simulink model "MdXX_DoneChk"  (R2024b)
settings: Solver=FixedStepDiscrete  StartTime=0.0  StopTime=10.0  FixedStep=0.01  RelTol=1e-3
undefined symbols (not defined in the file or in its folder): KeSMSuVehicleModelConfig_Val
libraries: simulink x44
(part 3 of 3)

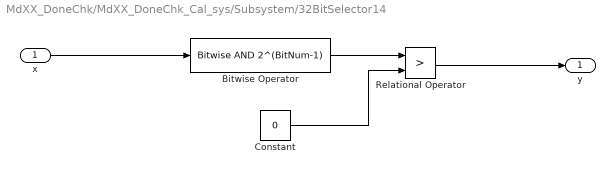
== system MdXX_DoneChk/MdXX_DoneChk_Cal_sys/Subsystem/32BitSelector14 ==
  x : Inport
  Bitwise Operator : simulink/Logic and Bit Operations/Bitwise Operator  logicop=AND  UseBitMask=on  BitMask=2^(BitNum-1)  BitMaskRealWorld=Stored Integer
  Constant : Constant  Value=0  OutDataTypeStr=uint32
  Relational Operator : RelationalOperator  Operator=>  OutDataTypeStr=boolean  RndMeth=Simplest  InputSameDT=off
  y : Outport  VectorParamsAs1DForOutWhenUnconnected=off
  wires:
  Relational Operator/1 -> y/1
  Constant/1 -> Relational Operator/2
  x/1 -> Bitwise Operator/1
  Bitwise Operator/1 -> Relational Operator/1

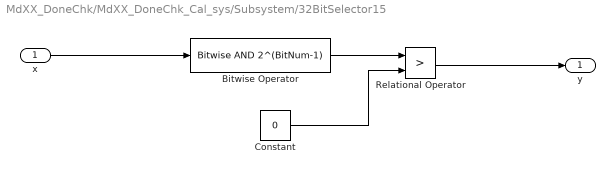
== system MdXX_DoneChk/MdXX_DoneChk_Cal_sys/Subsystem/32BitSelector15 ==
  x : Inport
  Bitwise Operator : simulink/Logic and Bit Operations/Bitwise Operator  logicop=AND  UseBitMask=on  BitMask=2^(BitNum-1)  BitMaskRealWorld=Stored Integer
  Constant : Constant  Value=0  OutDataTypeStr=uint32
  Relational Operator : RelationalOperator  Operator=>  OutDataTypeStr=boolean  RndMeth=Simplest  InputSameDT=off
  y : Outport  VectorParamsAs1DForOutWhenUnconnected=off
  wires:
  Bitwise Operator/1 -> Relational Operator/1
  x/1 -> Bitwise Operator/1
  Constant/1 -> Relational Operator/2
  Relational Operator/1 -> y/1

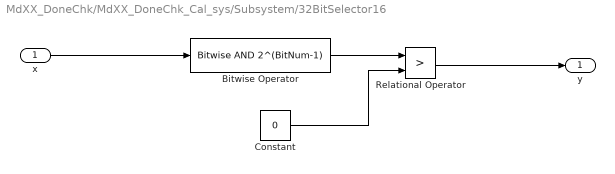
== system MdXX_DoneChk/MdXX_DoneChk_Cal_sys/Subsystem/32BitSelector16 ==
  x : Inport
  Bitwise Operator : simulink/Logic and Bit Operations/Bitwise Operator  logicop=AND  UseBitMask=on  BitMask=2^(BitNum-1)  BitMaskRealWorld=Stored Integer
  Constant : Constant  Value=0  OutDataTypeStr=uint32
  Relational Operator : RelationalOperator  Operator=>  OutDataTypeStr=boolean  RndMeth=Simplest  InputSameDT=off
  y : Outport  VectorParamsAs1DForOutWhenUnconnected=off
  wires:
  Relational Operator/1 -> y/1
  Constant/1 -> Relational Operator/2
  x/1 -> Bitwise Operator/1
  Bitwise Operator/1 -> Relational Operator/1

== system MdXX_DoneChk/MdXX_DoneChk_Cal_sys/Subsystem/32BitSelector17 ==
  x : Inport
  Bitwise Operator : simulink/Logic and Bit Operations/Bitwise Operator  logicop=AND  UseBitMask=on  BitMask=2^(BitNum-1)  BitMaskRealWorld=Stored Integer
  Constant : Constant  Value=0  OutDataTypeStr=uint32
  Relational Operator : RelationalOperator  Operator=>  OutDataTypeStr=boolean  RndMeth=Simplest  InputSameDT=off
  y : Outport  VectorParamsAs1DForOutWhenUnconnected=off
  wires:
  Bitwise Operator/1 -> Relational Operator/1
  x/1 -> Bitwise Operator/1
  Constant/1 -> Relational Operator/2
  Relational Operator/1 -> y/1

== system MdXX_DoneChk/MdXX_DoneChk_Cal_sys/Subsystem/32BitSelector18 ==
  x : Inport
  Bitwise Operator : simulink/Logic and Bit Operations/Bitwise Operator  logicop=AND  UseBitMask=on  BitMask=2^(BitNum-1)  BitMaskRealWorld=Stored Integer
  Constant : Constant  Value=0  OutDataTypeStr=uint32
  Relational Operator : RelationalOperator  Operator=>  OutDataTypeStr=boolean  RndMeth=Simplest  InputSameDT=off
  y : Outport  VectorParamsAs1DForOutWhenUnconnected=off
  wires:
  Relational Operator/1 -> y/1
  Constant/1 -> Relational Operator/2
  x/1 -> Bitwise Operator/1
  Bitwise Operator/1 -> Relational Operator/1

== system MdXX_DoneChk/MdXX_DoneChk_Cal_sys/Subsystem/32BitSelector19 ==
  x : Inport
  Bitwise Operator : simulink/Logic and Bit Operations/Bitwise Operator  logicop=AND  UseBitMask=on  BitMask=2^(BitNum-1)  BitMaskRealWorld=Stored Integer
  Constant : Constant  Value=0  OutDataTypeStr=uint32
  Relational Operator : RelationalOperator  Operator=>  OutDataTypeStr=boolean  RndMeth=Simplest  InputSameDT=off
  y : Outport  VectorParamsAs1DForOutWhenUnconnected=off
  wires:
  Bitwise Operator/1 -> Relational Operator/1
  x/1 -> Bitwise Operator/1
  Constant/1 -> Relational Operator/2
  Relational Operator/1 -> y/1

== system MdXX_DoneChk/MdXX_DoneChk_Cal_sys/Subsystem/32BitSelector2 ==
  x : Inport
  Bitwise Operator : simulink/Logic and Bit Operations/Bitwise Operator  logicop=AND  UseBitMask=on  BitMask=2^(BitNum-1)  BitMaskRealWorld=Stored Integer
  Constant : Constant  Value=0  OutDataTypeStr=uint32
  Relational Operator : RelationalOperator  Operator=>  OutDataTypeStr=boolean  RndMeth=Simplest  InputSameDT=off
  y : Outport  VectorParamsAs1DForOutWhenUnconnected=off
  wires:
  Relational Operator/1 -> y/1
  Constant/1 -> Relational Operator/2
  x/1 -> Bitwise Operator/1
  Bitwise Operator/1 -> Relational Operator/1

== system MdXX_DoneChk/MdXX_DoneChk_Cal_sys/Subsystem/32BitSelector20 ==
  x : Inport
  Bitwise Operator : simulink/Logic and Bit Operations/Bitwise Operator  logicop=AND  UseBitMask=on  BitMask=2^(BitNum-1)  BitMaskRealWorld=Stored Integer
  Constant : Constant  Value=0  OutDataTypeStr=uint32
  Relational Operator : RelationalOperator  Operator=>  OutDataTypeStr=boolean  RndMeth=Simplest  InputSameDT=off
  y : Outport  VectorParamsAs1DForOutWhenUnconnected=off
  wires:
  Relational Operator/1 -> y/1
  Constant/1 -> Relational Operator/2
  x/1 -> Bitwise Operator/1
  Bitwise Operator/1 -> Relational Operator/1

== system MdXX_DoneChk/MdXX_DoneChk_Cal_sys/Subsystem/32BitSelector21 ==
  x : Inport
  Bitwise Operator : simulink/Logic and Bit Operations/Bitwise Operator  logicop=AND  UseBitMask=on  BitMask=2^(BitNum-1)  BitMaskRealWorld=Stored Integer
  Constant : Constant  Value=0  OutDataTypeStr=uint32
  Relational Operator : RelationalOperator  Operator=>  OutDataTypeStr=boolean  RndMeth=Simplest  InputSameDT=off
  y : Outport  VectorParamsAs1DForOutWhenUnconnected=off
  wires:
  Bitwise Operator/1 -> Relational Operator/1
  x/1 -> Bitwise Operator/1
  Constant/1 -> Relational Operator/2
  Relational Operator/1 -> y/1

== system MdXX_DoneChk/MdXX_DoneChk_Cal_sys/Subsystem/32BitSelector22 ==
  x : Inport
  Bitwise Operator : simulink/Logic and Bit Operations/Bitwise Operator  logicop=AND  UseBitMask=on  BitMask=2^(BitNum-1)  BitMaskRealWorld=Stored Integer
  Constant : Constant  Value=0  OutDataTypeStr=uint32
  Relational Operator : RelationalOperator  Operator=>  OutDataTypeStr=boolean  RndMeth=Simplest  InputSameDT=off
  y : Outport  VectorParamsAs1DForOutWhenUnconnected=off
  wires:
  Relational Operator/1 -> y/1
  Constant/1 -> Relational Operator/2
  x/1 -> Bitwise Operator/1
  Bitwise Operator/1 -> Relational Operator/1

== system MdXX_DoneChk/MdXX_DoneChk_Cal_sys/Subsystem/32BitSelector23 ==
  x : Inport
  Bitwise Operator : simulink/Logic and Bit Operations/Bitwise Operator  logicop=AND  UseBitMask=on  BitMask=2^(BitNum-1)  BitMaskRealWorld=Stored Integer
  Constant : Constant  Value=0  OutDataTypeStr=uint32
  Relational Operator : RelationalOperator  Operator=>  OutDataTypeStr=boolean  RndMeth=Simplest  InputSameDT=off
  y : Outport  VectorParamsAs1DForOutWhenUnconnected=off
  wires:
  Bitwise Operator/1 -> Relational Operator/1
  x/1 -> Bitwise Operator/1
  Constant/1 -> Relational Operator/2
  Relational Operator/1 -> y/1

== system MdXX_DoneChk/MdXX_DoneChk_Cal_sys/Subsystem/32BitSelector24 ==
  x : Inport
  Bitwise Operator : simulink/Logic and Bit Operations/Bitwise Operator  logicop=AND  UseBitMask=on  BitMask=2^(BitNum-1)  BitMaskRealWorld=Stored Integer
  Constant : Constant  Value=0  OutDataTypeStr=uint32
  Relational Operator : RelationalOperator  Operator=>  OutDataTypeStr=boolean  RndMeth=Simplest  InputSameDT=off
  y : Outport  VectorParamsAs1DForOutWhenUnconnected=off
  wires:
  Relational Operator/1 -> y/1
  Constant/1 -> Relational Operator/2
  x/1 -> Bitwise Operator/1
  Bitwise Operator/1 -> Relational Operator/1

== system MdXX_DoneChk/MdXX_DoneChk_Cal_sys/Subsystem/32BitSelector25 ==
  x : Inport
  Bitwise Operator : simulink/Logic and Bit Operations/Bitwise Operator  logicop=AND  UseBitMask=on  BitMask=2^(BitNum-1)  BitMaskRealWorld=Stored Integer
  Constant : Constant  Value=0  OutDataTypeStr=uint32
  Relational Operator : RelationalOperator  Operator=>  OutDataTypeStr=boolean  RndMeth=Simplest  InputSameDT=off
  y : Outport  VectorParamsAs1DForOutWhenUnconnected=off
  wires:
  Bitwise Operator/1 -> Relational Operator/1
  x/1 -> Bitwise Operator/1
  Constant/1 -> Relational Operator/2
  Relational Operator/1 -> y/1

== system MdXX_DoneChk/MdXX_DoneChk_Cal_sys/Subsystem/32BitSelector26 ==
  x : Inport
  Bitwise Operator : simulink/Logic and Bit Operations/Bitwise Operator  logicop=AND  UseBitMask=on  BitMask=2^(BitNum-1)  BitMaskRealWorld=Stored Integer
  Constant : Constant  Value=0  OutDataTypeStr=uint32
  Relational Operator : RelationalOperator  Operator=>  OutDataTypeStr=boolean  RndMeth=Simplest  InputSameDT=off
  y : Outport  VectorParamsAs1DForOutWhenUnconnected=off
  wires:
  Relational Operator/1 -> y/1
  Constant/1 -> Relational Operator/2
  x/1 -> Bitwise Operator/1
  Bitwise Operator/1 -> Relational Operator/1

== system MdXX_DoneChk/MdXX_DoneChk_Cal_sys/Subsystem/32BitSelector27 ==
  x : Inport
  Bitwise Operator : simulink/Logic and Bit Operations/Bitwise Operator  logicop=AND  UseBitMask=on  BitMask=2^(BitNum-1)  BitMaskRealWorld=Stored Integer
  Constant : Constant  Value=0  OutDataTypeStr=uint32
  Relational Operator : RelationalOperator  Operator=>  OutDataTypeStr=boolean  RndMeth=Simplest  InputSameDT=off
  y : Outport  VectorParamsAs1DForOutWhenUnconnected=off
  wires:
  Bitwise Operator/1 -> Relational Operator/1
  x/1 -> Bitwise Operator/1
  Constant/1 -> Relational Operator/2
  Relational Operator/1 -> y/1

== system MdXX_DoneChk/MdXX_DoneChk_Cal_sys/Subsystem/32BitSelector28 ==
  x : Inport
  Bitwise Operator : simulink/Logic and Bit Operations/Bitwise Operator  logicop=AND  UseBitMask=on  BitMask=2^(BitNum-1)  BitMaskRealWorld=Stored Integer
  Constant : Constant  Value=0  OutDataTypeStr=uint32
  Relational Operator : RelationalOperator  Operator=>  OutDataTypeStr=boolean  RndMeth=Simplest  InputSameDT=off
  y : Outport  VectorParamsAs1DForOutWhenUnconnected=off
  wires:
  Relational Operator/1 -> y/1
  Constant/1 -> Relational Operator/2
  x/1 -> Bitwise Operator/1
  Bitwise Operator/1 -> Relational Operator/1

== system MdXX_DoneChk/MdXX_DoneChk_Cal_sys/Subsystem/32BitSelector29 ==
  x : Inport
  Bitwise Operator : simulink/Logic and Bit Operations/Bitwise Operator  logicop=AND  UseBitMask=on  BitMask=2^(BitNum-1)  BitMaskRealWorld=Stored Integer
  Constant : Constant  Value=0  OutDataTypeStr=uint32
  Relational Operator : RelationalOperator  Operator=>  OutDataTypeStr=boolean  RndMeth=Simplest  InputSameDT=off
  y : Outport  VectorParamsAs1DForOutWhenUnconnected=off
  wires:
  Bitwise Operator/1 -> Relational Operator/1
  x/1 -> Bitwise Operator/1
  Constant/1 -> Relational Operator/2
  Relational Operator/1 -> y/1

== system MdXX_DoneChk/MdXX_DoneChk_Cal_sys/Subsystem/32BitSelector3 ==
  x : Inport
  Bitwise Operator : simulink/Logic and Bit Operations/Bitwise Operator  logicop=AND  UseBitMask=on  BitMask=2^(BitNum-1)  BitMaskRealWorld=Stored Integer
  Constant : Constant  Value=0  OutDataTypeStr=uint32
  Relational Operator : RelationalOperator  Operator=>  OutDataTypeStr=boolean  RndMeth=Simplest  InputSameDT=off
  y : Outport  VectorParamsAs1DForOutWhenUnconnected=off
  wires:
  Bitwise Operator/1 -> Relational Operator/1
  x/1 -> Bitwise Operator/1
  Constant/1 -> Relational Operator/2
  Relational Operator/1 -> y/1

== system MdXX_DoneChk/MdXX_DoneChk_Cal_sys/Subsystem/32BitSelector30 ==
  x : Inport
  Bitwise Operator : simulink/Logic and Bit Operations/Bitwise Operator  logicop=AND  UseBitMask=on  BitMask=2^(BitNum-1)  BitMaskRealWorld=Stored Integer
  Constant : Constant  Value=0  OutDataTypeStr=uint32
  Relational Operator : RelationalOperator  Operator=>  OutDataTypeStr=boolean  RndMeth=Simplest  InputSameDT=off
  y : Outport  VectorParamsAs1DForOutWhenUnconnected=off
  wires:
  Relational Operator/1 -> y/1
  Constant/1 -> Relational Operator/2
  x/1 -> Bitwise Operator/1
  Bitwise Operator/1 -> Relational Operator/1

== system MdXX_DoneChk/MdXX_DoneChk_Cal_sys/Subsystem/32BitSelector31 ==
  x : Inport
  Bitwise Operator : simulink/Logic and Bit Operations/Bitwise Operator  logicop=AND  UseBitMask=on  BitMask=2^(BitNum-1)  BitMaskRealWorld=Stored Integer
  Constant : Constant  Value=0  OutDataTypeStr=uint32
  Relational Operator : RelationalOperator  Operator=>  OutDataTypeStr=boolean  RndMeth=Simplest  InputSameDT=off
  y : Outport  VectorParamsAs1DForOutWhenUnconnected=off
  wires:
  Relational Operator/1 -> y/1
  Constant/1 -> Relational Operator/2
  x/1 -> Bitwise Operator/1
  Bitwise Operator/1 -> Relational Operator/1

== system MdXX_DoneChk/MdXX_DoneChk_Cal_sys/Subsystem/32BitSelector32 ==
  x : Inport
  Bitwise Operator : simulink/Logic and Bit Operations/Bitwise Operator  logicop=AND  UseBitMask=on  BitMask=2^(BitNum-1)  BitMaskRealWorld=Stored Integer
  Constant : Constant  Value=0  OutDataTypeStr=uint32
  Relational Operator : RelationalOperator  Operator=>  OutDataTypeStr=boolean  RndMeth=Simplest  InputSameDT=off
  y : Outport  VectorParamsAs1DForOutWhenUnconnected=off
  wires:
  Relational Operator/1 -> y/1
  Constant/1 -> Relational Operator/2
  x/1 -> Bitwise Operator/1
  Bitwise Operator/1 -> Relational Operator/1

== system MdXX_DoneChk/MdXX_DoneChk_Cal_sys/Subsystem/32BitSelector33 ==
  x : Inport
  Bitwise Operator : simulink/Logic and Bit Operations/Bitwise Operator  logicop=AND  UseBitMask=on  BitMask=2^(BitNum-1)  BitMaskRealWorld=Stored Integer
  Constant : Constant  Value=0  OutDataTypeStr=uint32
  Relational Operator : RelationalOperator  Operator=>  OutDataTypeStr=boolean  RndMeth=Simplest  InputSameDT=off
  y : Outport  VectorParamsAs1DForOutWhenUnconnected=off
  wires:
  Bitwise Operator/1 -> Relational Operator/1
  x/1 -> Bitwise Operator/1
  Constant/1 -> Relational Operator/2
  Relational Operator/1 -> y/1

== system MdXX_DoneChk/MdXX_DoneChk_Cal_sys/Subsystem/32BitSelector34 ==
  x : Inport
  Bitwise Operator : simulink/Logic and Bit Operations/Bitwise Operator  logicop=AND  UseBitMask=on  BitMask=2^(BitNum-1)  BitMaskRealWorld=Stored Integer
  Constant : Constant  Value=0  OutDataTypeStr=uint32
  Relational Operator : RelationalOperator  Operator=>  OutDataTypeStr=boolean  RndMeth=Simplest  InputSameDT=off
  y : Outport  VectorParamsAs1DForOutWhenUnconnected=off
  wires:
  Relational Operator/1 -> y/1
  Constant/1 -> Relational Operator/2
  x/1 -> Bitwise Operator/1
  Bitwise Operator/1 -> Relational Operator/1

== system MdXX_DoneChk/MdXX_DoneChk_Cal_sys/Subsystem/32BitSelector35 ==
  x : Inport
  Bitwise Operator : simulink/Logic and Bit Operations/Bitwise Operator  logicop=AND  UseBitMask=on  BitMask=2^(BitNum-1)  BitMaskRealWorld=Stored Integer
  Constant : Constant  Value=0  OutDataTypeStr=uint32
  Relational Operator : RelationalOperator  Operator=>  OutDataTypeStr=boolean  RndMeth=Simplest  InputSameDT=off
  y : Outport  VectorParamsAs1DForOutWhenUnconnected=off
  wires:
  Bitwise Operator/1 -> Relational Operator/1
  x/1 -> Bitwise Operator/1
  Constant/1 -> Relational Operator/2
  Relational Operator/1 -> y/1

== system MdXX_DoneChk/MdXX_DoneChk_Cal_sys/Subsystem/32BitSelector36 ==
  x : Inport
  Bitwise Operator : simulink/Logic and Bit Operations/Bitwise Operator  logicop=AND  UseBitMask=on  BitMask=2^(BitNum-1)  BitMaskRealWorld=Stored Integer
  Constant : Constant  Value=0  OutDataTypeStr=uint32
  Relational Operator : RelationalOperator  Operator=>  OutDataTypeStr=boolean  RndMeth=Simplest  InputSameDT=off
  y : Outport  VectorParamsAs1DForOutWhenUnconnected=off
  wires:
  Bitwise Operator/1 -> Relational Operator/1
  x/1 -> Bitwise Operator/1
  Constant/1 -> Relational Operator/2
  Relational Operator/1 -> y/1

== system MdXX_DoneChk/MdXX_DoneChk_Cal_sys/Subsystem/32BitSelector37 ==
  x : Inport
  Bitwise Operator : simulink/Logic and Bit Operations/Bitwise Operator  logicop=AND  UseBitMask=on  BitMask=2^(BitNum-1)  BitMaskRealWorld=Stored Integer
  Constant : Constant  Value=0  OutDataTypeStr=uint32
  Relational Operator : RelationalOperator  Operator=>  OutDataTypeStr=boolean  RndMeth=Simplest  InputSameDT=off
  y : Outport  VectorParamsAs1DForOutWhenUnconnected=off
  wires:
  Relational Operator/1 -> y/1
  Constant/1 -> Relational Operator/2
  x/1 -> Bitwise Operator/1
  Bitwise Operator/1 -> Relational Operator/1

== system MdXX_DoneChk/MdXX_DoneChk_Cal_sys/Subsystem/32BitSelector38 ==
  x : Inport
  Bitwise Operator : simulink/Logic and Bit Operations/Bitwise Operator  logicop=AND  UseBitMask=on  BitMask=2^(BitNum-1)  BitMaskRealWorld=Stored Integer
  Constant : Constant  Value=0  OutDataTypeStr=uint32
  Relational Operator : RelationalOperator  Operator=>  OutDataTypeStr=boolean  RndMeth=Simplest  InputSameDT=off
  y : Outport  VectorParamsAs1DForOutWhenUnconnected=off
  wires:
  Bitwise Operator/1 -> Relational Operator/1
  x/1 -> Bitwise Operator/1
  Constant/1 -> Relational Operator/2
  Relational Operator/1 -> y/1

== system MdXX_DoneChk/MdXX_DoneChk_Cal_sys/Subsystem/32BitSelector39 ==
  x : Inport
  Bitwise Operator : simulink/Logic and Bit Operations/Bitwise Operator  logicop=AND  UseBitMask=on  BitMask=2^(BitNum-1)  BitMaskRealWorld=Stored Integer
  Constant : Constant  Value=0  OutDataTypeStr=uint32
  Relational Operator : RelationalOperator  Operator=>  OutDataTypeStr=boolean  RndMeth=Simplest  InputSameDT=off
  y : Outport  VectorParamsAs1DForOutWhenUnconnected=off
  wires:
  Bitwise Operator/1 -> Relational Operator/1
  x/1 -> Bitwise Operator/1
  Constant/1 -> Relational Operator/2
  Relational Operator/1 -> y/1

== system MdXX_DoneChk/MdXX_DoneChk_Cal_sys/Subsystem/32BitSelector4 ==
  x : Inport
  Bitwise Operator : simulink/Logic and Bit Operations/Bitwise Operator  logicop=AND  UseBitMask=on  BitMask=2^(BitNum-1)  BitMaskRealWorld=Stored Integer
  Constant : Constant  Value=0  OutDataTypeStr=uint32
  Relational Operator : RelationalOperator  Operator=>  OutDataTypeStr=boolean  RndMeth=Simplest  InputSameDT=off
  y : Outport  VectorParamsAs1DForOutWhenUnconnected=off
  wires:
  Relational Operator/1 -> y/1
  Constant/1 -> Relational Operator/2
  x/1 -> Bitwise Operator/1
  Bitwise Operator/1 -> Relational Operator/1

== system MdXX_DoneChk/MdXX_DoneChk_Cal_sys/Subsystem/32BitSelector5 ==
  x : Inport
  Bitwise Operator : simulink/Logic and Bit Operations/Bitwise Operator  logicop=AND  UseBitMask=on  BitMask=2^(BitNum-1)  BitMaskRealWorld=Stored Integer
  Constant : Constant  Value=0  OutDataTypeStr=uint32
  Relational Operator : RelationalOperator  Operator=>  OutDataTypeStr=boolean  RndMeth=Simplest  InputSameDT=off
  y : Outport  VectorParamsAs1DForOutWhenUnconnected=off
  wires:
  Bitwise Operator/1 -> Relational Operator/1
  x/1 -> Bitwise Operator/1
  Constant/1 -> Relational Operator/2
  Relational Operator/1 -> y/1

== system MdXX_DoneChk/MdXX_DoneChk_Cal_sys/Subsystem/32BitSelector6 ==
  x : Inport
  Bitwise Operator : simulink/Logic and Bit Operations/Bitwise Operator  logicop=AND  UseBitMask=on  BitMask=2^(BitNum-1)  BitMaskRealWorld=Stored Integer
  Constant : Constant  Value=0  OutDataTypeStr=uint32
  Relational Operator : RelationalOperator  Operator=>  OutDataTypeStr=boolean  RndMeth=Simplest  InputSameDT=off
  y : Outport  VectorParamsAs1DForOutWhenUnconnected=off
  wires:
  Relational Operator/1 -> y/1
  Constant/1 -> Relational Operator/2
  x/1 -> Bitwise Operator/1
  Bitwise Operator/1 -> Relational Operator/1

== system MdXX_DoneChk/MdXX_DoneChk_Cal_sys/Subsystem/32BitSelector7 ==
  x : Inport
  Bitwise Operator : simulink/Logic and Bit Operations/Bitwise Operator  logicop=AND  UseBitMask=on  BitMask=2^(BitNum-1)  BitMaskRealWorld=Stored Integer
  Constant : Constant  Value=0  OutDataTypeStr=uint32
  Relational Operator : RelationalOperator  Operator=>  OutDataTypeStr=boolean  RndMeth=Simplest  InputSameDT=off
  y : Outport  VectorParamsAs1DForOutWhenUnconnected=off
  wires:
  Bitwise Operator/1 -> Relational Operator/1
  x/1 -> Bitwise Operator/1
  Constant/1 -> Relational Operator/2
  Relational Operator/1 -> y/1

== system MdXX_DoneChk/MdXX_DoneChk_Cal_sys/Subsystem/32BitSelector8 ==
  x : Inport
  Bitwise Operator : simulink/Logic and Bit Operations/Bitwise Operator  logicop=AND  UseBitMask=on  BitMask=2^(BitNum-1)  BitMaskRealWorld=Stored Integer
  Constant : Constant  Value=0  OutDataTypeStr=uint32
  Relational Operator : RelationalOperator  Operator=>  OutDataTypeStr=boolean  RndMeth=Simplest  InputSameDT=off
  y : Outport  VectorParamsAs1DForOutWhenUnconnected=off
  wires:
  Relational Operator/1 -> y/1
  Constant/1 -> Relational Operator/2
  x/1 -> Bitwise Operator/1
  Bitwise Operator/1 -> Relational Operator/1

== system MdXX_DoneChk/MdXX_DoneChk_Cal_sys/Subsystem/32BitSelector9 ==
  x : Inport
  Bitwise Operator : simulink/Logic and Bit Operations/Bitwise Operator  logicop=AND  UseBitMask=on  BitMask=2^(BitNum-1)  BitMaskRealWorld=Stored Integer
  Constant : Constant  Value=0  OutDataTypeStr=uint32
  Relational Operator : RelationalOperator  Operator=>  OutDataTypeStr=boolean  RndMeth=Simplest  InputSameDT=off
  y : Outport  VectorParamsAs1DForOutWhenUnconnected=off
  wires:
  Bitwise Operator/1 -> Relational Operator/1
  x/1 -> Bitwise Operator/1
  Constant/1 -> Relational Operator/2
  Relational Operator/1 -> y/1

== system MdXX_DoneChk/MdXX_DoneChk_Cal_sys/Subsystem/Subsystem ==
  MdDone : Inport
  MdEn : Inport  Port=2
  Constant : Constant  Value=0  OutDataTypeStr=uint8
  Switch : Switch  Criteria=u2 > Threshold  SaturateOnIntegerOverflow=off  InputSameDT=off
  MdDoneOut : Outport  VectorParamsAs1DForOutWhenUnconnected=off
  wires:
  MdEn/1 -> Switch/2
  Switch/1 -> MdDoneOut/1
  MdDone/1 -> Switch/1
  Constant/1 -> Switch/3

== system MdXX_DoneChk/MdXX_DoneChk_Cal_sys/Subsystem/Subsystem1 ==
  MdDone : Inport
  MdEn : Inport  Port=2
  Constant : Constant  Value=0  OutDataTypeStr=uint8
  Switch : Switch  Criteria=u2 > Threshold  SaturateOnIntegerOverflow=off  InputSameDT=off
  MdDoneOut : Outport  VectorParamsAs1DForOutWhenUnconnected=off
  wires:
  Constant/1 -> Switch/3
  MdDone/1 -> Switch/1
  Switch/1 -> MdDoneOut/1
  MdEn/1 -> Switch/2

== system MdXX_DoneChk/MdXX_DoneChk_Cal_sys/Subsystem/Subsystem10 ==
  MdDone : Inport
  MdEn : Inport  Port=2
  Constant : Constant  Value=0  OutDataTypeStr=uint8
  Switch : Switch  Criteria=u2 > Threshold  SaturateOnIntegerOverflow=off  InputSameDT=off
  MdDoneOut : Outport  VectorParamsAs1DForOutWhenUnconnected=off
  wires:
  MdEn/1 -> Switch/2
  Switch/1 -> MdDoneOut/1
  MdDone/1 -> Switch/1
  Constant/1 -> Switch/3

== system MdXX_DoneChk/MdXX_DoneChk_Cal_sys/Subsystem/Subsystem11 ==
  MdDone : Inport
  MdEn : Inport  Port=2
  Constant : Constant  Value=0  OutDataTypeStr=uint8
  Switch : Switch  Criteria=u2 > Threshold  SaturateOnIntegerOverflow=off  InputSameDT=off
  MdDoneOut : Outport  VectorParamsAs1DForOutWhenUnconnected=off
  wires:
  Constant/1 -> Switch/3
  MdDone/1 -> Switch/1
  Switch/1 -> MdDoneOut/1
  MdEn/1 -> Switch/2

== system MdXX_DoneChk/MdXX_DoneChk_Cal_sys/Subsystem/Subsystem12 ==
  MdDone : Inport
  MdEn : Inport  Port=2
  Constant : Constant  Value=0  OutDataTypeStr=uint8
  Switch : Switch  Criteria=u2 > Threshold  SaturateOnIntegerOverflow=off  InputSameDT=off
  MdDoneOut : Outport  VectorParamsAs1DForOutWhenUnconnected=off
  wires:
  MdEn/1 -> Switch/2
  Switch/1 -> MdDoneOut/1
  MdDone/1 -> Switch/1
  Constant/1 -> Switch/3

== system MdXX_DoneChk/MdXX_DoneChk_Cal_sys/Subsystem/Subsystem13 ==
  MdDone : Inport
  MdEn : Inport  Port=2
  Constant : Constant  Value=0  OutDataTypeStr=uint8
  Switch : Switch  Criteria=u2 > Threshold  SaturateOnIntegerOverflow=off  InputSameDT=off
  MdDoneOut : Outport  VectorParamsAs1DForOutWhenUnconnected=off
  wires:
  Constant/1 -> Switch/3
  MdDone/1 -> Switch/1
  Switch/1 -> MdDoneOut/1
  MdEn/1 -> Switch/2

== system MdXX_DoneChk/MdXX_DoneChk_Cal_sys/Subsystem/Subsystem14 ==
  MdDone : Inport
  MdEn : Inport  Port=2
  Constant : Constant  Value=0  OutDataTypeStr=uint8
  Switch : Switch  Criteria=u2 > Threshold  SaturateOnIntegerOverflow=off  InputSameDT=off
  MdDoneOut : Outport  VectorParamsAs1DForOutWhenUnconnected=off
  wires:
  MdEn/1 -> Switch/2
  Switch/1 -> MdDoneOut/1
  MdDone/1 -> Switch/1
  Constant/1 -> Switch/3

== system MdXX_DoneChk/MdXX_DoneChk_Cal_sys/Subsystem/Subsystem15 ==
  MdDone : Inport
  MdEn : Inport  Port=2
  Constant : Constant  Value=0  OutDataTypeStr=uint8
  Switch : Switch  Criteria=u2 > Threshold  SaturateOnIntegerOverflow=off  InputSameDT=off
  MdDoneOut : Outport  VectorParamsAs1DForOutWhenUnconnected=off
  wires:
  Constant/1 -> Switch/3
  MdDone/1 -> Switch/1
  Switch/1 -> MdDoneOut/1
  MdEn/1 -> Switch/2

== system MdXX_DoneChk/MdXX_DoneChk_Cal_sys/Subsystem/Subsystem16 ==
  MdDone : Inport
  MdEn : Inport  Port=2
  Constant : Constant  Value=0  OutDataTypeStr=uint8
  Switch : Switch  Criteria=u2 > Threshold  SaturateOnIntegerOverflow=off  InputSameDT=off
  MdDoneOut : Outport  VectorParamsAs1DForOutWhenUnconnected=off
  wires:
  MdEn/1 -> Switch/2
  Switch/1 -> MdDoneOut/1
  MdDone/1 -> Switch/1
  Constant/1 -> Switch/3

== system MdXX_DoneChk/MdXX_DoneChk_Cal_sys/Subsystem/Subsystem17 ==
  MdDone : Inport
  MdEn : Inport  Port=2
  Constant : Constant  Value=0  OutDataTypeStr=uint8
  Switch : Switch  Criteria=u2 > Threshold  SaturateOnIntegerOverflow=off  InputSameDT=off
  MdDoneOut : Outport  VectorParamsAs1DForOutWhenUnconnected=off
  wires:
  Constant/1 -> Switch/3
  MdDone/1 -> Switch/1
  Switch/1 -> MdDoneOut/1
  MdEn/1 -> Switch/2

== system MdXX_DoneChk/MdXX_DoneChk_Cal_sys/Subsystem/Subsystem18 ==
  MdDone : Inport
  MdEn : Inport  Port=2
  Constant : Constant  Value=0  OutDataTypeStr=uint8
  Switch : Switch  Criteria=u2 > Threshold  SaturateOnIntegerOverflow=off  InputSameDT=off
  MdDoneOut : Outport  VectorParamsAs1DForOutWhenUnconnected=off
  wires:
  MdEn/1 -> Switch/2
  Switch/1 -> MdDoneOut/1
  MdDone/1 -> Switch/1
  Constant/1 -> Switch/3

== system MdXX_DoneChk/MdXX_DoneChk_Cal_sys/Subsystem/Subsystem19 ==
  MdDone : Inport
  MdEn : Inport  Port=2
  Constant : Constant  Value=0  OutDataTypeStr=uint8
  Switch : Switch  Criteria=u2 > Threshold  SaturateOnIntegerOverflow=off  InputSameDT=off
  MdDoneOut : Outport  VectorParamsAs1DForOutWhenUnconnected=off
  wires:
  Constant/1 -> Switch/3
  MdDone/1 -> Switch/1
  Switch/1 -> MdDoneOut/1
  MdEn/1 -> Switch/2

== system MdXX_DoneChk/MdXX_DoneChk_Cal_sys/Subsystem/Subsystem2 ==
  MdDone : Inport
  MdEn : Inport  Port=2
  Constant : Constant  Value=0  OutDataTypeStr=uint8
  Switch : Switch  Criteria=u2 > Threshold  SaturateOnIntegerOverflow=off  InputSameDT=off
  MdDoneOut : Outport  VectorParamsAs1DForOutWhenUnconnected=off
  wires:
  MdEn/1 -> Switch/2
  Switch/1 -> MdDoneOut/1
  MdDone/1 -> Switch/1
  Constant/1 -> Switch/3

== system MdXX_DoneChk/MdXX_DoneChk_Cal_sys/Subsystem/Subsystem20 ==
  MdDone : Inport
  MdEn : Inport  Port=2
  Constant : Constant  Value=0  OutDataTypeStr=uint8
  Switch : Switch  Criteria=u2 > Threshold  SaturateOnIntegerOverflow=off  InputSameDT=off
  MdDoneOut : Outport  VectorParamsAs1DForOutWhenUnconnected=off
  wires:
  MdEn/1 -> Switch/2
  Switch/1 -> MdDoneOut/1
  MdDone/1 -> Switch/1
  Constant/1 -> Switch/3

== system MdXX_DoneChk/MdXX_DoneChk_Cal_sys/Subsystem/Subsystem21 ==
  MdDone : Inport
  MdEn : Inport  Port=2
  Constant : Constant  Value=0  OutDataTypeStr=uint8
  Switch : Switch  Criteria=u2 > Threshold  SaturateOnIntegerOverflow=off  InputSameDT=off
  MdDoneOut : Outport  VectorParamsAs1DForOutWhenUnconnected=off
  wires:
  Constant/1 -> Switch/3
  MdDone/1 -> Switch/1
  Switch/1 -> MdDoneOut/1
  MdEn/1 -> Switch/2

== system MdXX_DoneChk/MdXX_DoneChk_Cal_sys/Subsystem/Subsystem22 ==
  MdDone : Inport
  MdEn : Inport  Port=2
  Constant : Constant  Value=0  OutDataTypeStr=uint8
  Switch : Switch  Criteria=u2 > Threshold  SaturateOnIntegerOverflow=off  InputSameDT=off
  MdDoneOut : Outport  VectorParamsAs1DForOutWhenUnconnected=off
  wires:
  MdEn/1 -> Switch/2
  Switch/1 -> MdDoneOut/1
  MdDone/1 -> Switch/1
  Constant/1 -> Switch/3

== system MdXX_DoneChk/MdXX_DoneChk_Cal_sys/Subsystem/Subsystem23 ==
  MdDone : Inport
  MdEn : Inport  Port=2
  Constant : Constant  Value=0  OutDataTypeStr=uint8
  Switch : Switch  Criteria=u2 > Threshold  SaturateOnIntegerOverflow=off  InputSameDT=off
  MdDoneOut : Outport  VectorParamsAs1DForOutWhenUnconnected=off
  wires:
  Constant/1 -> Switch/3
  MdDone/1 -> Switch/1
  Switch/1 -> MdDoneOut/1
  MdEn/1 -> Switch/2

== system MdXX_DoneChk/MdXX_DoneChk_Cal_sys/Subsystem/Subsystem24 ==
  MdDone : Inport
  MdEn : Inport  Port=2
  Constant : Constant  Value=0  OutDataTypeStr=uint8
  Switch : Switch  Criteria=u2 > Threshold  SaturateOnIntegerOverflow=off  InputSameDT=off
  MdDoneOut : Outport  VectorParamsAs1DForOutWhenUnconnected=off
  wires:
  MdEn/1 -> Switch/2
  Switch/1 -> MdDoneOut/1
  MdDone/1 -> Switch/1
  Constant/1 -> Switch/3

== system MdXX_DoneChk/MdXX_DoneChk_Cal_sys/Subsystem/Subsystem25 ==
  MdDone : Inport
  MdEn : Inport  Port=2
  Constant : Constant  Value=0  OutDataTypeStr=uint8
  Switch : Switch  Criteria=u2 > Threshold  SaturateOnIntegerOverflow=off  InputSameDT=off
  MdDoneOut : Outport  VectorParamsAs1DForOutWhenUnconnected=off
  wires:
  Constant/1 -> Switch/3
  MdDone/1 -> Switch/1
  Switch/1 -> MdDoneOut/1
  MdEn/1 -> Switch/2

== system MdXX_DoneChk/MdXX_DoneChk_Cal_sys/Subsystem/Subsystem26 ==
  MdDone : Inport
  MdEn : Inport  Port=2
  Constant : Constant  Value=0  OutDataTypeStr=uint8
  Switch : Switch  Criteria=u2 > Threshold  SaturateOnIntegerOverflow=off  InputSameDT=off
  MdDoneOut : Outport  VectorParamsAs1DForOutWhenUnconnected=off
  wires:
  MdEn/1 -> Switch/2
  Switch/1 -> MdDoneOut/1
  MdDone/1 -> Switch/1
  Constant/1 -> Switch/3

== system MdXX_DoneChk/MdXX_DoneChk_Cal_sys/Subsystem/Subsystem27 ==
  MdDone : Inport
  MdEn : Inport  Port=2
  Constant : Constant  Value=0  OutDataTypeStr=uint8
  Switch : Switch  Criteria=u2 > Threshold  SaturateOnIntegerOverflow=off  InputSameDT=off
  MdDoneOut : Outport  VectorParamsAs1DForOutWhenUnconnected=off
  wires:
  Constant/1 -> Switch/3
  MdDone/1 -> Switch/1
  Switch/1 -> MdDoneOut/1
  MdEn/1 -> Switch/2

== system MdXX_DoneChk/MdXX_DoneChk_Cal_sys/Subsystem/Subsystem28 ==
  MdDone : Inport
  MdEn : Inport  Port=2
  Constant : Constant  Value=0  OutDataTypeStr=uint8
  Switch : Switch  Criteria=u2 > Threshold  SaturateOnIntegerOverflow=off  InputSameDT=off
  MdDoneOut : Outport  VectorParamsAs1DForOutWhenUnconnected=off
  wires:
  MdEn/1 -> Switch/2
  Switch/1 -> MdDoneOut/1
  MdDone/1 -> Switch/1
  Constant/1 -> Switch/3

== system MdXX_DoneChk/MdXX_DoneChk_Cal_sys/Subsystem/Subsystem29 ==
  MdDone : Inport
  MdEn : Inport  Port=2
  Constant : Constant  Value=0  OutDataTypeStr=uint8
  Switch : Switch  Criteria=u2 > Threshold  SaturateOnIntegerOverflow=off  InputSameDT=off
  MdDoneOut : Outport  VectorParamsAs1DForOutWhenUnconnected=off
  wires:
  Constant/1 -> Switch/3
  MdDone/1 -> Switch/1
  Switch/1 -> MdDoneOut/1
  MdEn/1 -> Switch/2

== system MdXX_DoneChk/MdXX_DoneChk_Cal_sys/Subsystem/Subsystem3 ==
  MdDone : Inport
  MdEn : Inport  Port=2
  Constant : Constant  Value=0  OutDataTypeStr=uint8
  Switch : Switch  Criteria=u2 > Threshold  SaturateOnIntegerOverflow=off  InputSameDT=off
  MdDoneOut : Outport  VectorParamsAs1DForOutWhenUnconnected=off
  wires:
  Constant/1 -> Switch/3
  MdDone/1 -> Switch/1
  Switch/1 -> MdDoneOut/1
  MdEn/1 -> Switch/2

== system MdXX_DoneChk/MdXX_DoneChk_Cal_sys/Subsystem/Subsystem30 ==
  MdDone : Inport
  MdEn : Inport  Port=2
  Constant : Constant  Value=0  OutDataTypeStr=uint8
  Switch : Switch  Criteria=u2 > Threshold  SaturateOnIntegerOverflow=off  InputSameDT=off
  MdDoneOut : Outport  VectorParamsAs1DForOutWhenUnconnected=off
  wires:
  MdEn/1 -> Switch/2
  Switch/1 -> MdDoneOut/1
  MdDone/1 -> Switch/1
  Constant/1 -> Switch/3

== system MdXX_DoneChk/MdXX_DoneChk_Cal_sys/Subsystem/Subsystem31 ==
  MdDone : Inport
  MdEn : Inport  Port=2
  Constant : Constant  Value=0  OutDataTypeStr=uint8
  Switch : Switch  Criteria=u2 > Threshold  SaturateOnIntegerOverflow=off  InputSameDT=off
  MdDoneOut : Outport  VectorParamsAs1DForOutWhenUnconnected=off
  wires:
  MdEn/1 -> Switch/2
  Switch/1 -> MdDoneOut/1
  MdDone/1 -> Switch/1
  Constant/1 -> Switch/3

== system MdXX_DoneChk/MdXX_DoneChk_Cal_sys/Subsystem/Subsystem4 ==
  MdDone : Inport
  MdEn : Inport  Port=2
  Constant : Constant  Value=0  OutDataTypeStr=uint8
  Switch : Switch  Criteria=u2 > Threshold  SaturateOnIntegerOverflow=off  InputSameDT=off
  MdDoneOut : Outport  VectorParamsAs1DForOutWhenUnconnected=off
  wires:
  MdEn/1 -> Switch/2
  Switch/1 -> MdDoneOut/1
  MdDone/1 -> Switch/1
  Constant/1 -> Switch/3

== system MdXX_DoneChk/MdXX_DoneChk_Cal_sys/Subsystem/Subsystem5 ==
  MdDone : Inport
  MdEn : Inport  Port=2
  Constant : Constant  Value=0  OutDataTypeStr=uint8
  Switch : Switch  Criteria=u2 > Threshold  SaturateOnIntegerOverflow=off  InputSameDT=off
  MdDoneOut : Outport  VectorParamsAs1DForOutWhenUnconnected=off
  wires:
  Constant/1 -> Switch/3
  MdDone/1 -> Switch/1
  Switch/1 -> MdDoneOut/1
  MdEn/1 -> Switch/2

== system MdXX_DoneChk/MdXX_DoneChk_Cal_sys/Subsystem/Subsystem6 ==
  MdDone : Inport
  MdEn : Inport  Port=2
  Constant : Constant  Value=0  OutDataTypeStr=uint8
  Switch : Switch  Criteria=u2 > Threshold  SaturateOnIntegerOverflow=off  InputSameDT=off
  MdDoneOut : Outport  VectorParamsAs1DForOutWhenUnconnected=off
  wires:
  MdEn/1 -> Switch/2
  Switch/1 -> MdDoneOut/1
  MdDone/1 -> Switch/1
  Constant/1 -> Switch/3

== system MdXX_DoneChk/MdXX_DoneChk_Cal_sys/Subsystem/Subsystem7 ==
  MdDone : Inport
  MdEn : Inport  Port=2
  Constant : Constant  Value=0  OutDataTypeStr=uint8
  Switch : Switch  Criteria=u2 > Threshold  SaturateOnIntegerOverflow=off  InputSameDT=off
  MdDoneOut : Outport  VectorParamsAs1DForOutWhenUnconnected=off
  wires:
  Constant/1 -> Switch/3
  MdDone/1 -> Switch/1
  Switch/1 -> MdDoneOut/1
  MdEn/1 -> Switch/2

== system MdXX_DoneChk/MdXX_DoneChk_Cal_sys/Subsystem/Subsystem8 ==
  MdDone : Inport
  MdEn : Inport  Port=2
  Constant : Constant  Value=0  OutDataTypeStr=uint8
  Switch : Switch  Criteria=u2 > Threshold  SaturateOnIntegerOverflow=off  InputSameDT=off
  MdDoneOut : Outport  VectorParamsAs1DForOutWhenUnconnected=off
  wires:
  MdEn/1 -> Switch/2
  Switch/1 -> MdDoneOut/1
  MdDone/1 -> Switch/1
  Constant/1 -> Switch/3

== system MdXX_DoneChk/MdXX_DoneChk_Cal_sys/Subsystem/Subsystem9 ==
  MdDone : Inport
  MdEn : Inport  Port=2
  Constant : Constant  Value=0  OutDataTypeStr=uint8
  Switch : Switch  Criteria=u2 > Threshold  SaturateOnIntegerOverflow=off  InputSameDT=off
  MdDoneOut : Outport  VectorParamsAs1DForOutWhenUnconnected=off
  wires:
  Constant/1 -> Switch/3
  MdDone/1 -> Switch/1
  Switch/1 -> MdDoneOut/1
  MdEn/1 -> Switch/2
